simulink model "simulation"  (R2016a)
settings: Solver=VariableStepAuto  StartTime=0.0  StopTime=100  FixedStep=0.01  MaxStep=0.01  RelTol=1e-3
values from neighbouring files (symbols this model uses):
  g = 9.81    [main.m]
  kdp = 15    [main.m]
  kdps = 15    [main.m]
  kdt = 15    [main.m]
  kdx = 1    [main.m]
  kdz = 20    [main.m]
  kpp = 100    [main.m]
  kpps = 100    [main.m]
  kpt = 100    [main.m]
  kpx = 1.05    [main.m]
  kpz = 100    [main.m]
  m = 0.65    [main.m]
  r_rel_1 = r_rel_but    [create_r_relative.m]
  r_rel_2 = r_rel_circle    [create_r_relative.m]
  r_rel_3 = r_rel_line    [create_r_relative.m]
  xi_init = zeros(6,N)    [main.m]
undefined symbols (not defined in the file or in its folder): A_c, A_c_2
libraries: simulink x2
settings Model: Creator=Jens  LastModifiedBy=Jens

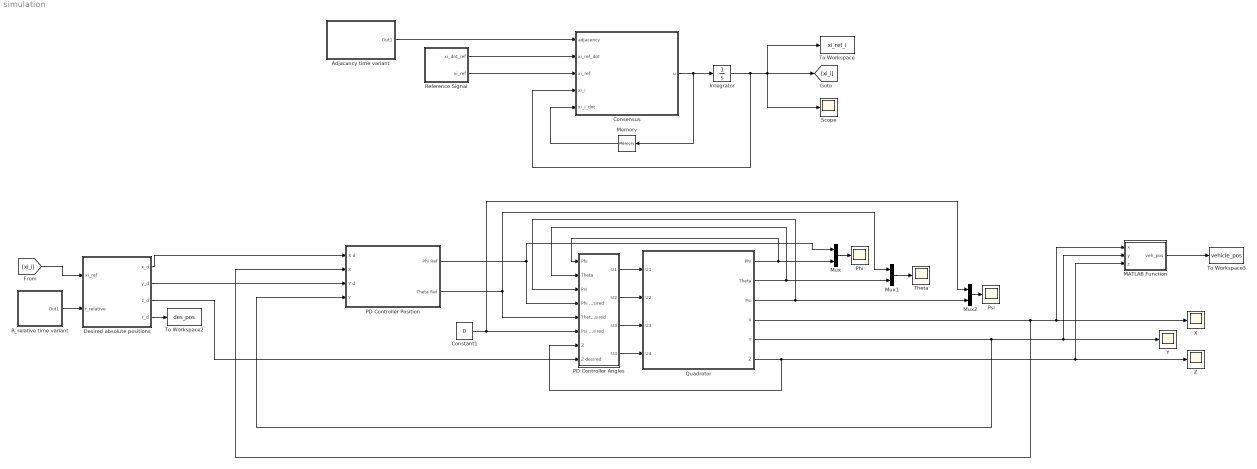
== system simulation ==
  Adjacancy time variant : Subsystem
  Consensus : MATLAB Function  TreatAsAtomicUnit=on
      settings: MinAlgLoopOccurrences=on
  Constant1 : Constant  Value=0
  Desired absolute positions : MATLAB Function  TreatAsAtomicUnit=on
  Integrator : Integrator  InitialCondition=xi_init
  MATLAB Function : MATLAB Function  TreatAsAtomicUnit=on
  Memory : Memory
  Mux : Mux  Inputs=2
  Mux1 : Mux  Inputs=2
  Mux2 : Mux  Inputs=2
  PD Controller Angles : Subsystem
  PD Controller Position : Subsystem
  Phi : Scope
  Psi : Scope
  Quadrotor : Subsystem
  R_relative time variant : Subsystem
  Reference Signal : Subsystem
  Scope : Scope
  Theta : Scope
  To Workspace : ToWorkspace  VariableName=xi_ref_i  SaveFormat=Timeseries  SampleTime=-1
  To Workspace2 : ToWorkspace  VariableName=des_pos  SaveFormat=Timeseries  SampleTime=-1
  To Workspace3 : ToWorkspace  VariableName=vehicle_pos  SaveFormat=Timeseries  SampleTime=-1
  X : Scope
  Y : Scope
  Z : Scope
  wires:
  Integrator/1 -> Scope/1, [xi_i], To Workspace/1, Consensus/4(xi_i)
  Consensus/1(u) -> Integrator/1, Memory/1
  Memory/1 -> Consensus/5(xi_i_dot)
  [xi_i] -> Desired absolute positions/1(xi_ref)
  Reference Signal/1(xi_dot_ref) -> Consensus/2(xi_ref_dot)
  Reference Signal/2(xi_ref) -> Consensus/3(xi_ref)
  Adjacancy time variant/1(Out1) -> Consensus/1(adjacency)
  R_relative time variant/1(Out1) -> Desired absolute positions/2(r_relative)
  PD Controller Angles/1(U1) -> Quadrotor/1(U1)
  PD Controller Angles/2(U2) -> Quadrotor/2(U2)
  PD Controller Angles/3(U3) -> Quadrotor/3(U3)
  PD Controller Angles/4(U4) -> Quadrotor/4(U4)
  Quadrotor/1(Phi) -> PD Controller Angles/1(Phi), Mux/2
  Quadrotor/2(Theta) -> PD Controller Angles/2(Theta), Mux1/2
  Quadrotor/3(Psi) -> PD Controller Angles/3(Psi), Mux2/2
  PD Controller Position/1(Phi Ref) -> PD Controller Angles/4(Phi desired), Mux/1
  PD Controller Position/2(Theta Ref) -> PD Controller Angles/5(Theta desired), Mux1/1
  Constant1/1 -> Mux2/1, PD Controller Angles/6(Psi desired)
  Desired absolute positions/3(z_d) -> PD Controller Angles/8(Z desired)
  Quadrotor/5(Y) -> PD Controller Position/4(Y), Y/1, MATLAB Function/2(y)
  Quadrotor/4(X) -> MATLAB Function/1(x), X/1, PD Controller Position/2(X)
  Mux/1 -> Phi/1
  Mux1/1 -> Theta/1
  Mux2/1 -> Psi/1
  Quadrotor/6(Z) -> PD Controller Angles/7(Z), Z/1, MATLAB Function/3(z)
  Desired absolute positions/2(y_d) -> PD Controller Position/3(Y d)
  Desired absolute positions/1(x_d) -> PD Controller Position/1(X d)
  MATLAB Function/1(veh_pos) -> To Workspace3/1
  Desired absolute positions/4(r_d) -> To Workspace2/1

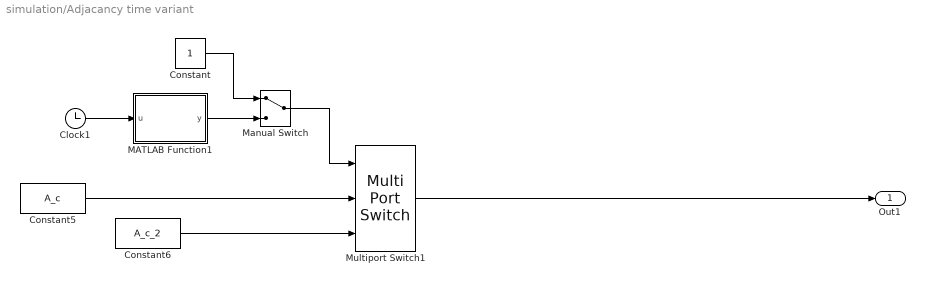
== system simulation/Adjacancy time variant ==
  Clock1 : Clock
  Constant : Constant
  Constant5 : Constant  Value=A_c
  Constant6 : Constant  Value=A_c_2
  MATLAB Function1 : MATLAB Function  TreatAsAtomicUnit=on
  Manual Switch : ManualSwitch
  Multiport Switch1 : MultiPortSwitch  Inputs=2
  Out1 : Outport
  wires:
  Manual Switch/1 -> Multiport Switch1/1
  Clock1/1 -> MATLAB Function1/1(u)
  Multiport Switch1/1 -> Out1/1
  Constant6/1 -> Multiport Switch1/3
  Constant5/1 -> Multiport Switch1/2
  Constant/1 -> Manual Switch/1
  MATLAB Function1/1(y) -> Manual Switch/2

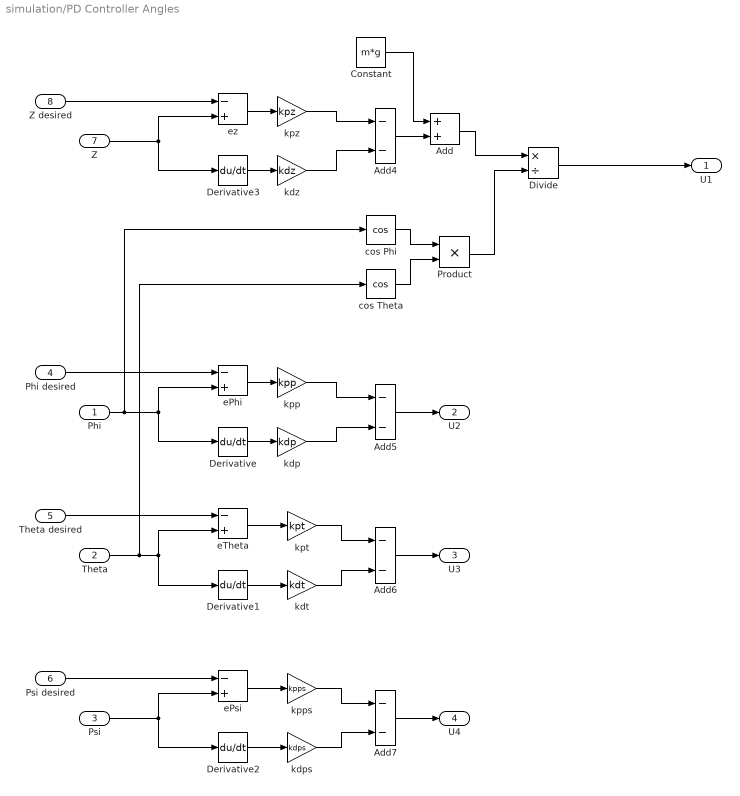
== system simulation/PD Controller Angles ==
  Phi : Inport
  Theta : Inport  Port=2
  Psi : Inport  Port=3
  Phi desired : Inport  Port=4
  Theta desired : Inport  Port=5
  Psi desired : Inport  Port=6
  Z : Inport  Port=7
  Z desired : Inport  Port=8
  Add : Sum
  Add{4..7} (4 alike) : Sum  Inputs=--
  Constant : Constant  Value=m*g
  Derivative{,1..3} (4 alike) : Derivative
  Divide : Product  Inputs=*/
  Product : Product  RndMeth=Zero
  cos Phi : Trigonometry  Operator=cos
  cos Theta : Trigonometry  Operator=cos
  ePhi : Sum  Inputs=-+
  ePsi : Sum  Inputs=-+
  eTheta : Sum  Inputs=-+
  ez : Sum  Inputs=-+
  kdp : Gain  Gain=kdp
  kdps : Gain  Gain=kdps
  kdt : Gain  Gain=kdt
  kdz : Gain  Gain=kdz
  kpp : Gain  Gain=kpp
  kpps : Gain  Gain=kpps
  kpt : Gain  Gain=kpt
  kpz : Gain  Gain=kpz
  U1 : Outport
  U2 : Outport  Port=2
  U3 : Outport  Port=3
  U4 : Outport  Port=4
  wires:
  Phi/1 -> Derivative/1, ePhi/2, cos Phi/1
  Theta/1 -> Derivative1/1, eTheta/2, cos Theta/1
  Psi/1 -> Derivative2/1, ePsi/2
  Phi desired/1 -> ePhi/1
  Theta desired/1 -> eTheta/1
  Psi desired/1 -> ePsi/1
  ePhi/1 -> kpp/1
  Derivative/1 -> kdp/1
  eTheta/1 -> kpt/1
  Derivative1/1 -> kdt/1
  ePsi/1 -> kpps/1
  Derivative2/1 -> kdps/1
  Z/1 -> Derivative3/1, ez/2
  Z desired/1 -> ez/1
  ez/1 -> kpz/1
  Derivative3/1 -> kdz/1
  kpz/1 -> Add4/1
  kdz/1 -> Add4/2
  kpp/1 -> Add5/1
  kdp/1 -> Add5/2
  Add5/1 -> U2/1
  kpt/1 -> Add6/1
  kdt/1 -> Add6/2
  Add6/1 -> U3/1
  kpps/1 -> Add7/1
  kdps/1 -> Add7/2
  Add7/1 -> U4/1
  cos Phi/1 -> Product/1
  cos Theta/1 -> Product/2
  Add4/1 -> Add/2
  Add/1 -> Divide/1
  Product/1 -> Divide/2
  Divide/1 -> U1/1
  Constant/1 -> Add/1

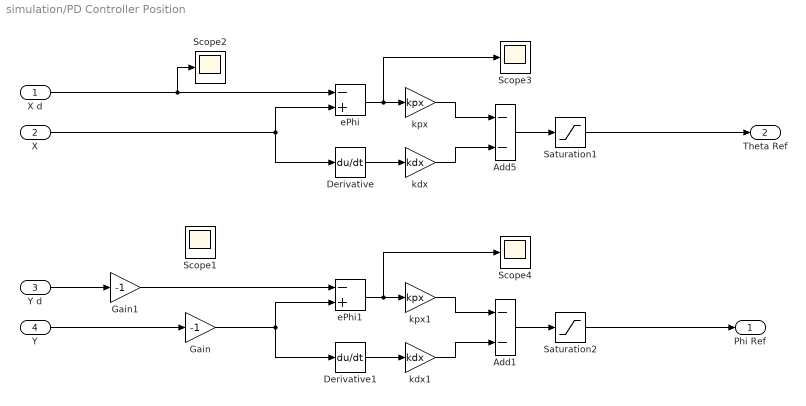
== system simulation/PD Controller Position ==
  X d : Inport
  X : Inport  Port=2
  Y d : Inport  Port=3
  Y : Inport  Port=4
  Add1 : Sum  Inputs=--
  Add5 : Sum  Inputs=--
  Derivative : Derivative
  Derivative1 : Derivative
  Gain : Gain  Gain=-1
  Gain1 : Gain  Gain=-1
  Saturation1 : Saturate  UpperLimit=0.05  LowerLimit=-0.05  ZeroCross=off
  Saturation2 : Saturate  UpperLimit=0.05  LowerLimit=-0.05  ZeroCross=off
  Scope{1..4} (4 alike) : Scope
  ePhi : Sum  Inputs=-+
  ePhi1 : Sum  Inputs=-+
  kdx : Gain  Gain=kdx
  kdx1 : Gain  Gain=kdx
  kpx : Gain  Gain=kpx
  kpx1 : Gain  Gain=kpx
  Phi Ref : Outport
  Theta Ref : Outport  Port=2
  wires:
  X/1 -> Derivative/1, ePhi/2
  X d/1 -> Scope2/1, ePhi/1
  ePhi/1 -> Scope3/1, kpx/1
  Derivative/1 -> kdx/1
  kpx/1 -> Add5/1
  kdx/1 -> Add5/2
  Add5/1 -> Saturation1/1
  Gain/1 -> Derivative1/1, ePhi1/2
  ePhi1/1 -> Scope4/1, kpx1/1
  Derivative1/1 -> kdx1/1
  kpx1/1 -> Add1/1
  kdx1/1 -> Add1/2
  Add1/1 -> Saturation2/1
  Saturation2/1 -> Phi Ref/1
  Y/1 -> Gain/1
  Saturation1/1 -> Theta Ref/1
  Y d/1 -> Gain1/1
  Gain1/1 -> ePhi1/1

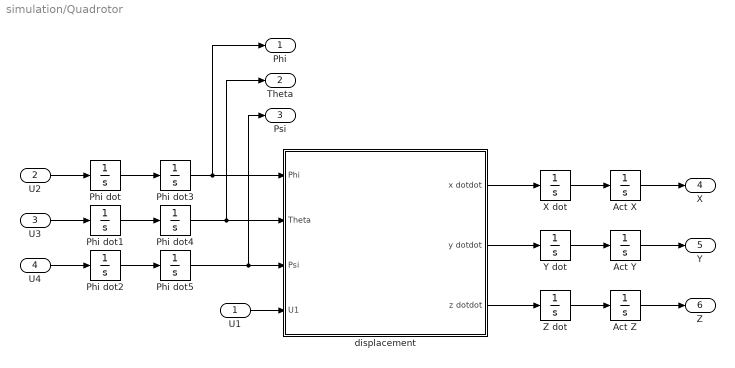
== system simulation/Quadrotor ==
  U1 : Inport
  U2 : Inport  Port=2
  U3 : Inport  Port=3
  U4 : Inport  Port=4
  Act X : Integrator
  Act Y : Integrator
  Act Z : Integrator
  Phi dot : Integrator
  Phi dot{1..5} (5 alike) : Integrator  ZeroCross=off
  X dot : Integrator
  Y dot : Integrator
  Z dot : Integrator
  displacement : Subsystem
  Phi : Outport
  Theta : Outport  Port=2
  Psi : Outport  Port=3
  X : Outport  Port=4
  Y : Outport  Port=5
  Z : Outport  Port=6
  wires:
  U2/1 -> Phi dot/1
  U3/1 -> Phi dot1/1
  U4/1 -> Phi dot2/1
  Phi dot/1 -> Phi dot3/1
  Phi dot1/1 -> Phi dot4/1
  Phi dot2/1 -> Phi dot5/1
  Phi dot3/1 -> displacement/1(Phi), Phi/1
  Phi dot4/1 -> displacement/2(Theta), Theta/1
  Phi dot5/1 -> Psi/1, displacement/3(Psi)
  displacement/1(x dotdot) -> X dot/1
  X dot/1 -> Act X/1
  Y dot/1 -> Act Y/1
  displacement/2(y dotdot) -> Y dot/1
  Z dot/1 -> Act Z/1
  displacement/3(z dotdot) -> Z dot/1
  Act X/1 -> X/1
  Act Y/1 -> Y/1
  Act Z/1 -> Z/1
  U1/1 -> displacement/4(U1)

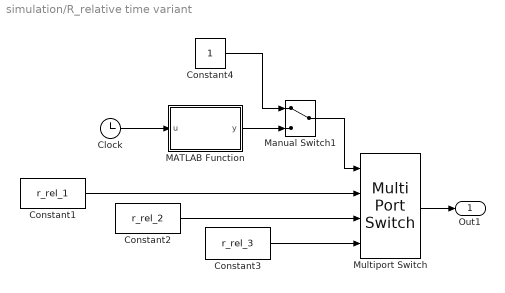
== system simulation/R_relative time variant ==
  Clock : Clock
  Constant1 : Constant  Value=r_rel_1
  Constant2 : Constant  Value=r_rel_2
  Constant3 : Constant  Value=r_rel_3
  Constant4 : Constant
  MATLAB Function : MATLAB Function  TreatAsAtomicUnit=on
  Manual Switch1 : ManualSwitch
  Multiport Switch : MultiPortSwitch
  Out1 : Outport
  wires:
  Constant4/1 -> Manual Switch1/1
  MATLAB Function/1(y) -> Manual Switch1/2
  Manual Switch1/1 -> Multiport Switch/1
  Constant1/1 -> Multiport Switch/2
  Constant2/1 -> Multiport Switch/3
  Clock/1 -> MATLAB Function/1(u)
  Multiport Switch/1 -> Out1/1
  Constant3/1 -> Multiport Switch/4

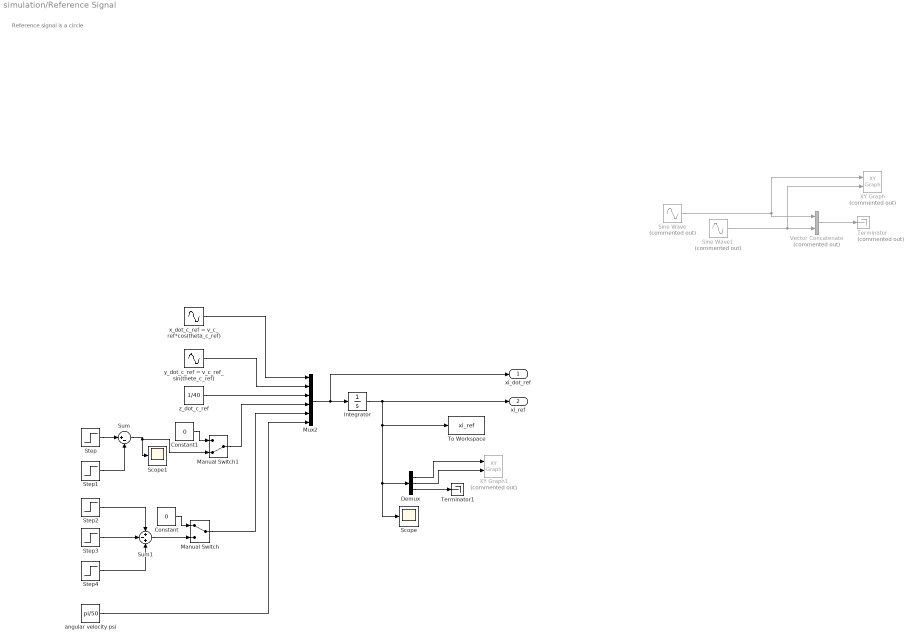
== system simulation/Reference Signal ==
  note: Reference signal is a circle
  Constant : Constant  Value=0
  Constant1 : Constant  Value=0
  Demux : Demux  Outputs=3
  Integrator : Integrator  InitialCondition=[0;0;0;0;0;0]
  Manual Switch : ManualSwitch
  Manual Switch1 : ManualSwitch  CurrentSetting=0
  Mux2 : Mux  Inputs=6
  Scope : Scope
  Scope1 : Scope
  Sine Wave : Sin  Commented=on  Phase=pi/2  SampleTime=0
  Sine Wave1 : Sin  Commented=on  SampleTime=0
  Step : Step  Time=20  After=pi/10  SampleTime=0
  Step1 : Step  Time=40  After=pi/10  SampleTime=0
  Step2 : Step  Time=10  After=pi/30  SampleTime=0
  Step3 : Step  Time=15  After=pi/30*2  SampleTime=0
  Step4 : Step  Time=20  After=pi/30  SampleTime=0
  Sum : Sum  Inputs=|+-
  Sum1 : Sum  Inputs=+-+
  Terminator : Terminator  Commented=on
  Terminator1 : Terminator
  To Workspace : ToWorkspace  VariableName=xi_ref  SaveFormat=Timeseries  SampleTime=-1
  Vector Concatenate : Concatenate  Commented=on
  XY Graph : simulink/Sinks/XY Graph  Commented=on  xmin=-1  xmax=1  ymin=-1  ymax=1  st=-1
  XY Graph1 : simulink/Sinks/XY Graph  Commented=on  xmin=-1  xmax=1  ymin=-1  ymax=3  st=-1
  angular velocity psi : Constant  Value=pi/50
  x_dot_c_ref = v_c_ref*cos(theta_c_ref) : Sin  Amplitude=9*pi/500  Frequency=pi/50  Phase=pi/2  SampleTime=0
  y_dot_c_ref = v_c_ref_sin(thete_c_ref) : Sin  Amplitude=9*pi/500  Frequency=pi/50  SampleTime=0
  z_dot_c_ref : Constant  Value=1/40
  xi_dot_ref : Outport
  xi_ref : Outport  Port=2
  wires:
  Sine Wave1/1 -> XY Graph/2, Vector Concatenate/2
  Sine Wave/1 -> Vector Concatenate/1, XY Graph/1
  Vector Concatenate/1 -> Terminator/1
  Demux/1 -> XY Graph1/1
  Demux/2 -> XY Graph1/2
  Demux/3 -> Terminator1/1
  y_dot_c_ref = v_c_ref_sin(thete_c_ref)/1 -> Mux2/2
  x_dot_c_ref = v_c_ref*cos(theta_c_ref)/1 -> Mux2/1
  Mux2/1 -> xi_dot_ref/1, Integrator/1
  Integrator/1 -> To Workspace/1, Scope/1, Demux/1, xi_ref/1
  angular velocity psi/1 -> Mux2/6
  z_dot_c_ref/1 -> Mux2/3
  Step/1 -> Sum/1
  Step1/1 -> Sum/2
  Step2/1 -> Sum1/1
  Step3/1 -> Sum1/2
  Step4/1 -> Sum1/3
  Sum1/1 -> Manual Switch/2
  Manual Switch/1 -> Mux2/5
  Constant/1 -> Manual Switch/1
  Sum/1 -> Manual Switch1/2, Scope1/1
  Constant1/1 -> Manual Switch1/1
  Manual Switch1/1 -> Mux2/4

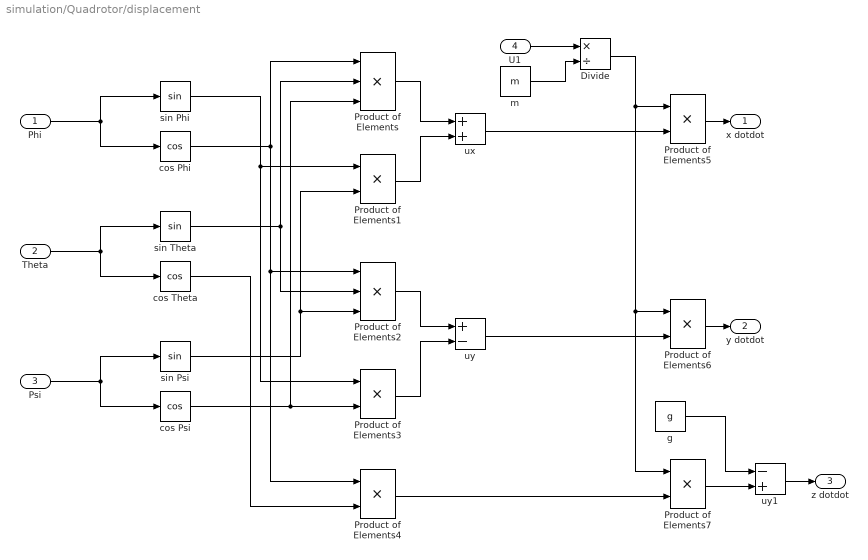
== system simulation/Quadrotor/displacement ==
  Phi : Inport
  Theta : Inport  Port=2
  Psi : Inport  Port=3
  U1 : Inport  Port=4
  Divide : Product  Inputs=*/
  Product of Elements : Product  Inputs=3
  Product of Elements{1,3..7} (6 alike) : Product
  Product of Elements2 : Product  Inputs=3
  cos Phi : Trigonometry  Operator=cos
  cos Psi : Trigonometry  Operator=cos
  cos Theta : Trigonometry  Operator=cos
  g : Constant  Value=g
  m : Constant  Value=m
  sin Phi : Trigonometry
  sin Psi : Trigonometry
  sin Theta : Trigonometry
  ux : Sum
  uy : Sum  Inputs=+-
  uy1 : Sum  Inputs=-+
  x dotdot : Outport
  y dotdot : Outport  Port=2
  z dotdot : Outport  Port=3
  wires:
  Phi/1 -> sin Phi/1, cos Phi/1
  Theta/1 -> sin Theta/1, cos Theta/1
  Psi/1 -> sin Psi/1, cos Psi/1
  sin Theta/1 -> Product of Elements/2, Product of Elements2/2
  cos Psi/1 -> Product of Elements/3, Product of Elements3/2
  cos Phi/1 -> Product of Elements/1, Product of Elements2/1, Product of Elements4/1
  sin Phi/1 -> Product of Elements1/1, Product of Elements3/1
  sin Psi/1 -> Product of Elements1/2, Product of Elements2/3
  Product of Elements/1 -> ux/1
  Product of Elements1/1 -> ux/2
  ux/1 -> Product of Elements5/2
  Product of Elements2/1 -> uy/1
  Product of Elements3/1 -> uy/2
  uy/1 -> Product of Elements6/2
  cos Theta/1 -> Product of Elements4/2
  Product of Elements4/1 -> Product of Elements7/2
  U1/1 -> Divide/1
  m/1 -> Divide/2
  Divide/1 -> Product of Elements5/1, Product of Elements6/1, Product of Elements7/1
  Product of Elements5/1 -> x dotdot/1
  Product of Elements6/1 -> y dotdot/1
  uy1/1 -> z dotdot/1
  Product of Elements7/1 -> uy1/2
  g/1 -> uy1/1

== matlab function simulation/Adjacancy time variant/MATLAB Function1 ==
  data: u input; y output
function y = fcn(u)

if (u >= 20 && u < 60)
    y = 2;
else
    y = 1;
end

== matlab function simulation/Consensus ==
  data: adjacency input; u output; xi_ref_dot input; xi_ref input; xi_i input; xi_i_dot input
function u = fcn(adjacency, xi_ref_dot, xi_ref, xi_i, xi_i_dot)
% calculates u = xi_i_dot for all vehicles according to the conensus
% formula for time-varying reference state (access to the leader only to a subgroup)

% Number of vehicles
N = size(adjacency,1)-1;
% initialize output u to zero
u = zeros(6,N);

% scalar to influence convergence speed
gamma = 1;

% formula to calculate xi_dot_i = u_i for each vehicle compare p. 196
% [REN08] formula 10.1
% u consists of six states per vehicle in a 6xN matrix / updates each
% vehicle after another (6 states per iteration of outer for loop)
for i=1:1:N
    eta = sum(adjacency(i,:));
    % if vehicle has no incoming connection (equal to eta = 0) u is set to zero therefore the
    % information states don't change and remain constant
    if (eta == 0)
        u(:,i) = zeros(6,1);
    else
        temp = zeros(6,1);
        for j=1:1:N
            temp = temp + adjacency(i,j)*(xi_i_dot(:,j)-gamma*(xi_i(:,i)-xi_i(:,j)));
        end
        u(:,i) = 1/eta * temp + 1/eta * adjacency(i,N+1)*(xi_ref_dot-gamma*(xi_i(:,i)-xi_ref));
    end    
end

== matlab function simulation/R_relative time variant/MATLAB Function ==
  data: u input; y output
function y = fcn(u)

if (u < 20)
    y = 1;
elseif (u >= 20 && u < 50)
    y = 2;
elseif (u >= 50 && u < 100)
    y = 3;
else
    y = 1;
end

== matlab function simulation/Desired absolute positions ==
  data: xi_ref input; x_d output; r_relative input; y_d output; z_d output; r_d output
function [x_d,y_d,z_d,r_d]  = desired_pos_abs(xi_ref, r_relative)
% desired_pos_abs computes the desired absolute positions depending on the
% reference frame of the vehicle and the relative coordinates of the desired positions
% outputs x_d and y_d in a vector r_d
% inputs are xi_ref = [x_coordinate_frame, y_coordinate_frame,
% theta_coordinate frame theta phi psi] the reference frame for each
% vehicle

% set matrix nxn
r_d = zeros(size(r_relative));



%loop over each vehicle
for i=1:1:size(r_relative,2)
    
    % infromation state of the vehicle angle
    psi = xi_ref(6,i);
    phi = xi_ref(5,i);
    theta = xi_ref(4,i);
    
    % Drehmatrix Dz
    Dz = [cos(psi) -sin(psi) 0
        sin(psi)  cos(psi) 0
        0   0    1];
    
    % Drehmatrix Dy
    Dy = [cos(phi)  0   sin(phi)
        0      1      0
        -sin(phi)  0   cos(phi)];
    
    % Drehmatrix Dx
    Dx = [1     0         0
        0  cos(theta) -sin(theta)
        0  sin(theta)  cos(theta)];
     
    r_d(:,i) = xi_ref(1:3,i) + Dz*Dy*Dx*r_relative(:,i);
end

x_d = r_d(1,:);
y_d = r_d(2,:);
z_d = r_d(3,:);

end

== matlab function simulation/MATLAB Function ==
  data: x input; veh_pos output; y input; z input
function veh_pos = fcn(x,y,z)
%#codegen

veh_pos = [x;y;z];
